simulink model "ICE_assignment"  (R2022a)
settings: Solver=FixedStepDiscrete  StartTime=0.0  StopTime=inf  RelTol=1e-3
undefined symbols (not defined in the file): Friend_Distance, Friend_Latitude, Friend_Longitude, My_Distance, My_Latitude, My_Longitude, sender
libraries: androidcommunicationlib x13, androiduilib x8, androidaudiovideolib x3, androidsensorlib x1
settings Model: Creator=GautamVashishtha  LastModifiedBy=GautamVashishtha
settings OptimizationCC: EnhancedBackFolding=on  PassReuseOutputArgsAs=Individual arguments  ZeroExternalMemoryAtStartup=off  ZeroInternalMemoryAtStartup=off  MaxStackSize=64  OptimizeBlockOrder=speed  DifferentSizesBufferReuse=on  OptimizationCustomize=off  EfficientTunableParamExpr=on
settings DebuggingCC: ParameterTunabilityLossMsg=error
settings HardwareCC: ProdBitPerPointer=32  ProdBitPerSizeT=32  ProdBitPerPtrDiffT=32  ProdLargestAtomicInteger=Long  ProdLargestAtomicFloat=Double  ProdWordSize=32  ProdHWDeviceType=ARM Compatible->ARM Cortex  UseEmbeddedCoderFeatures=off  UseSimulinkCoderFeatures=off
settings SFSimCC: MATLABDynamicMemAlloc=off
settings RTWCC: SystemTargetFile=ert.tlc  HardwareBoard=Android Device  TLCOptions="-aInlineSetEventsForThisBaseRateFcn=TLC_FALSE -aSuppressMultiTaskScheduler=TLC_FALSE  -aRateBasedStepFcn=0"  TemplateMakefile=ert_default_tmf  RTWVerbose=off  Toolchain=Android SDK/NDK Tools
settings CodeAppCC: ForceParamTrailComments=on  IgnoreCustomStorageClasses=off  OperatorAnnotations=on  SimulinkDataObjDesc=on  SFDataObjDesc=on  InsertBlockDesc=on
settings ERTTargetCC: SupportNonInlinedSFcns=on

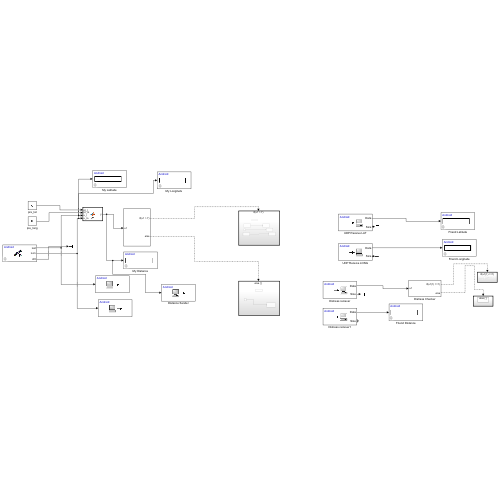
[thumbnail: Simulink's stored preview of the top-level diagram]
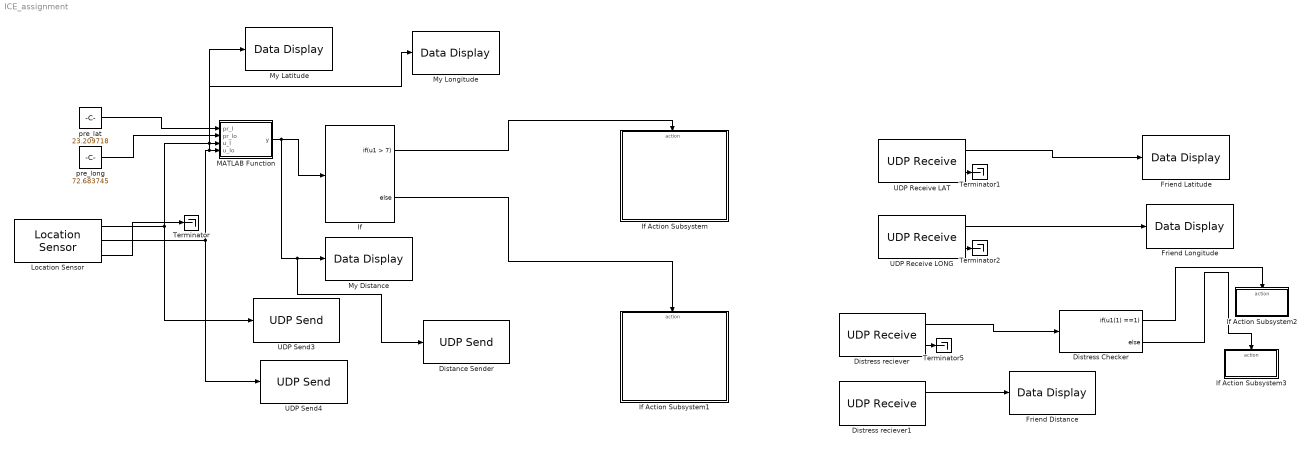
== system ICE_assignment ==
  Distance Sender : androidcommunicationlib/UDP Send  remoteURL='10.7.57.20'  remotePort=1234  localURL='0.0.0.0'  localPortSource=Automatically determine  localPort=-1  sampletime=-1  blockPlatform=Android  separateLengthPort=0
      settings: SourceProductBaseCode=ANDROID
  Distress Checker : If  IfExpression=u1(1) ==1
  Distress reciever : androidcommunicationlib/UDP Receive  localURL='0.0.0.0'  localPort=3000  remoteURL='0.0.0.0'  remotePort=-1  recvBufferSize=8192  signalDatatype=double  dims=1  isVarSize=off  showBlockingTime=off  blockingTime=0  sampletime=0.1  blockPlatform=Android
      settings: SourceProductBaseCode=ANDROID
  Distress reciever1 : androidcommunicationlib/UDP Receive  localURL='0.0.0.0'  localPort=1234  remoteURL='0.0.0.0'  remotePort=-1  recvBufferSize=8192  signalDatatype=double  dims=1  isVarSize=off  showBlockingTime=off  blockingTime=0  sampletime=0.1  blockPlatform=Android
      settings: SourceProductBaseCode=ANDROID
  Friend Distance : androiduilib/Data Display  DataDisplayId=sender/Friend_Distance  Format=Float  Precision=6  SimulateUsing=Code generation  blockPlatform=Android
      settings: SourceProductBaseCode=ANDROID
  Friend Latitude : androiduilib/Data Display  DataDisplayId=sender/Friend_Latitude  Format=Float  Precision=6  SimulateUsing=Code generation  blockPlatform=Android
      settings: SourceProductBaseCode=ANDROID
  Friend Longitude : androiduilib/Data Display  DataDisplayId=sender/Friend_Longitude  Format=Float  Precision=6  SimulateUsing=Code generation  blockPlatform=Android
      settings: SourceProductBaseCode=ANDROID
  If : If  IfExpression=u1 > 7
  If Action Subsystem : Subsystem  TreatAsAtomicUnit=on
  If Action Subsystem1 : Subsystem  TreatAsAtomicUnit=on
  If Action Subsystem2 : Subsystem  TreatAsAtomicUnit=on
  If Action Subsystem3 : Subsystem  TreatAsAtomicUnit=on
  Location Sensor : androidsensorlib/Location Sensor  OutputVector=off  SampleTime=10  BlockPlatform=Android
      settings: SourceProductBaseCode=ANDROID
  MATLAB Function : MATLAB Function  TreatAsAtomicUnit=on
  My Distance : androiduilib/Data Display  DataDisplayId=sender/My_Distance  Format=Float  Precision=6  SimulateUsing=Code generation  blockPlatform=Android
      settings: SourceProductBaseCode=ANDROID
  My Latitude : androiduilib/Data Display  DataDisplayId=sender/My_Latitude  Format=Float  Precision=6  SimulateUsing=Code generation  blockPlatform=Android
      settings: SourceProductBaseCode=ANDROID
  My Longitude : androiduilib/Data Display  DataDisplayId=sender/My_Longitude  Format=Float  Precision=6  SimulateUsing=Code generation  blockPlatform=Android
      settings: SourceProductBaseCode=ANDROID
  Terminator{,1..2,5} (4 alike) : Terminator
  UDP Receive LAT : androidcommunicationlib/UDP Receive  localURL='0.0.0.0'  localPort=5000  remoteURL='0.0.0.0'  remotePort=-1  recvBufferSize=8192  signalDatatype=double  dims=1  isVarSize=off  showBlockingTime=off  blockingTime=0  sampletime=0.1  blockPlatform=Android
      settings: SourceProductBaseCode=ANDROID
  UDP Receive LONG : androidcommunicationlib/UDP Receive  localURL='0.0.0.0'  localPort=4000  remoteURL='0.0.0.0'  remotePort=-1  recvBufferSize=8192  signalDatatype=double  dims=1  isVarSize=off  showBlockingTime=off  blockingTime=0  sampletime=0.1  blockPlatform=Android
      settings: SourceProductBaseCode=ANDROID
  UDP Send3 : androidcommunicationlib/UDP Send  remoteURL='10.7.57.20'  remotePort=5000  localURL='0.0.0.0'  localPortSource=Automatically determine  localPort=-1  sampletime=-1  blockPlatform=Android  separateLengthPort=0
      settings: SourceProductBaseCode=ANDROID
  UDP Send4 : androidcommunicationlib/UDP Send  remoteURL='10.7.57.20'  remotePort=4000  localURL='0.0.0.0'  localPortSource=Automatically determine  localPort=-1  sampletime=-1  blockPlatform=Android  separateLengthPort=0
      settings: SourceProductBaseCode=ANDROID
  pre_lat : Constant  Value=23.209718  SampleTime=0.1
  pre_long : Constant  Value=72.683745  SampleTime=0.1
  wires:
  Location Sensor/2 -> My Longitude/1, MATLAB Function/4(u_lo), UDP Send4/1
  MATLAB Function/1(y) -> Distance Sender/1, My Distance/1, If/1
  Location Sensor/3 -> Terminator/1
  pre_lat/1 -> MATLAB Function/1(pr_l)
  pre_long/1 -> MATLAB Function/2(pr_lo)
  Location Sensor/1 -> My Latitude/1, MATLAB Function/3(u_l), UDP Send3/1
  If/1 -> If Action Subsystem/Action
  If/2 -> If Action Subsystem1/Action
  UDP Receive LONG/1 -> Friend Longitude/1
  Distress reciever/1 -> Distress Checker/1
  Distress reciever/2 -> Terminator5/1
  UDP Receive LAT/1 -> Friend Latitude/1
  UDP Receive LAT/2 -> Terminator1/1
  UDP Receive LONG/2 -> Terminator2/1
  Distress Checker/1 -> If Action Subsystem2/Action
  Distress Checker/2 -> If Action Subsystem3/Action
  Distress reciever1/1 -> Friend Distance/1

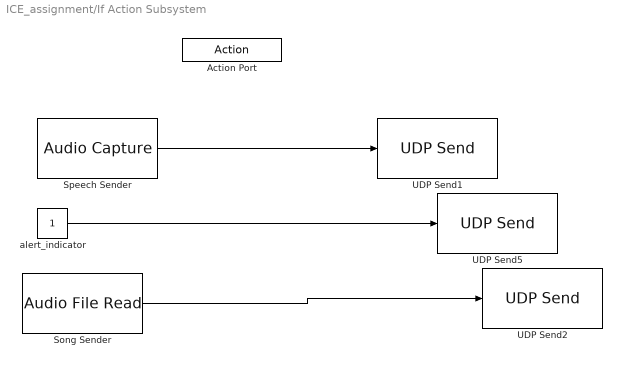
== system ICE_assignment/If Action Subsystem ==
  Action Port : ActionPort  ActionPortLabel=if(u1 > 7)
  Song Sender : androidaudiovideolib/Audio File Read  FileName=guitartune.wav  FrameSize=4410
      settings: SourceProductBaseCode=ANDROID
  Speech Sender : androidaudiovideolib/Audio Capture  SampleFreq=44100  FrameSize=4410  SampleTime=0.1  SimulateUsing=Code generation  DeviceStr=0  QueueDuration=0  BlockPlatform=Android  AudioSamplingFreq=44100
      settings: SourceProductBaseCode=ANDROID
  UDP Send1 : androidcommunicationlib/UDP Send  remoteURL='10.7.57.20'  remotePort=8000  localURL='0.0.0.0'  localPortSource=Automatically determine  localPort=-1  sampletime=-1  blockPlatform=Android  separateLengthPort=0
      settings: SourceProductBaseCode=ANDROID
  UDP Send2 : androidcommunicationlib/UDP Send  remoteURL='10.7.57.20'  remotePort=8001  localURL='0.0.0.0'  localPortSource=Automatically determine  localPort=-1  sampletime=-1  blockPlatform=Android  separateLengthPort=0
      settings: SourceProductBaseCode=ANDROID
  UDP Send5 : androidcommunicationlib/UDP Send  remoteURL='10.7.57.20'  remotePort=3000  localURL='0.0.0.0'  localPortSource=Automatically determine  localPort=-1  sampletime=-1  blockPlatform=Android  separateLengthPort=0
      settings: SourceProductBaseCode=ANDROID
  alert_indicator : Constant
  wires:
  Speech Sender/1 -> UDP Send1/1
  alert_indicator/1 -> UDP Send5/1
  Song Sender/1 -> UDP Send2/1

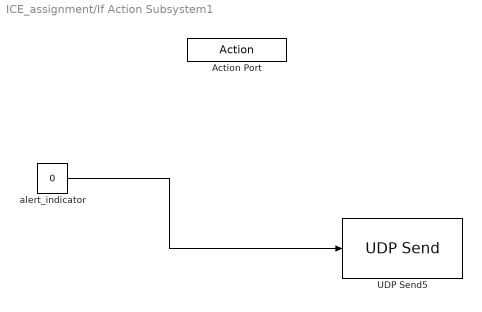
== system ICE_assignment/If Action Subsystem1 ==
  Action Port : ActionPort  ActionPortLabel=else
  UDP Send5 : androidcommunicationlib/UDP Send  remoteURL='10.7.57.20'  remotePort=3000  localURL='0.0.0.0'  localPortSource=Automatically determine  localPort=-1  sampletime=-1  blockPlatform=Android  separateLengthPort=0
      settings: SourceProductBaseCode=ANDROID
  alert_indicator : Constant  Value=0  SampleTime=0.1
  wires:
  alert_indicator/1 -> UDP Send5/1

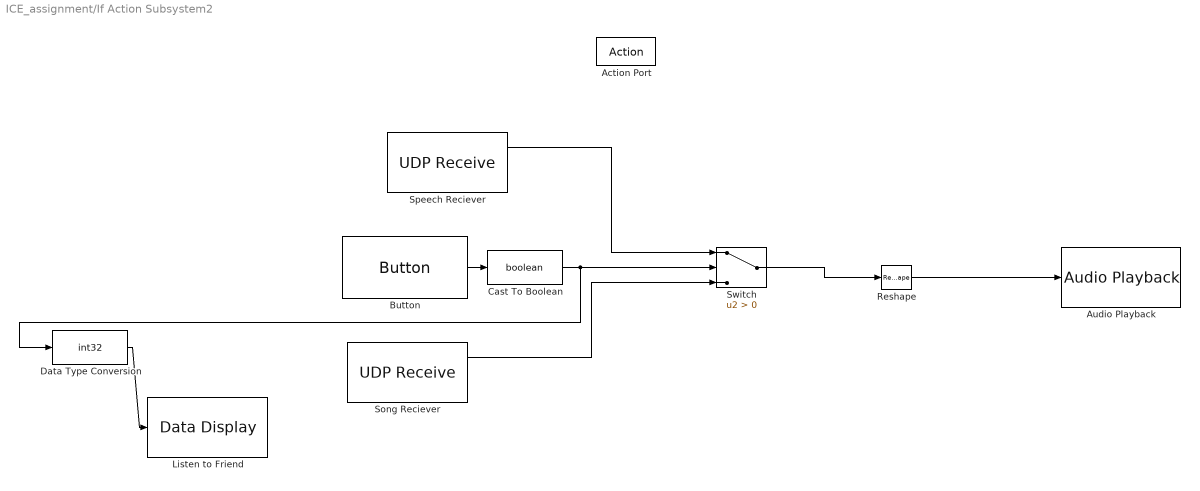
== system ICE_assignment/If Action Subsystem2 ==
  Action Port : ActionPort  ActionPortLabel=if(u1(1) ==1)
  Audio Playback : androidaudiovideolib/Audio Playback  SampleFreq=44100  AudioSamplingFreq=44100  SampleTime=0.1  DeviceStr=0  QueueDuration=0  BlockPlatform=Android
      settings: SourceProductBaseCode=ANDROID
  Button : androiduilib/Button  ButtonState=Not pressed  ButtonId=sender/If_Action_Subsystem2/Button  State=off  SampleTime=0.1  BlockPlatform=Android
      settings: SourceProductBaseCode=ANDROID
  Cast To Boolean : DataTypeConversion  OutDataTypeStr=boolean  SaturateOnIntegerOverflow=off  RndMeth=Floor
  Data Type Conversion : DataTypeConversion  OutDataTypeStr=int32  SaturateOnIntegerOverflow=off  RndMeth=Floor
  Listen to Friend : androiduilib/Data Display  DataDisplayId=sender/If_Action_Subsystem2/Listen_to_Friend  Format=Integer  Precision=6  SimulateUsing=Code generation  blockPlatform=Android
      settings: SourceProductBaseCode=ANDROID
  Reshape : Reshape  OutputDimensionality=Customize  OutputDimensions=[4410,2]
  Song Reciever : androidcommunicationlib/UDP Receive  localURL='0.0.0.0'  localPort=8001  remoteURL='0.0.0.0'  remotePort=-1  recvBufferSize=8192  signalDatatype=int16  dims=8820  isVarSize=off  showBlockingTime=off  blockingTime=0  sampletime=0.1  blockPlatform=Android
      settings: SourceProductBaseCode=ANDROID
  Speech Reciever : androidcommunicationlib/UDP Receive  localURL='0.0.0.0'  localPort=8000  remoteURL='0.0.0.0'  remotePort=-1  recvBufferSize=8192  signalDatatype=int16  dims=8820  isVarSize=off  showBlockingTime=off  blockingTime=0  sampletime=0.1  blockPlatform=Android
      settings: SourceProductBaseCode=ANDROID
  Switch : Switch  Criteria=u2 > Threshold  SaturateOnIntegerOverflow=off  InputSameDT=off
  wires:
  Reshape/1 -> Audio Playback/1
  Button/1 -> Cast To Boolean/1
  Speech Reciever/1 -> Switch/1
  Song Reciever/1 -> Switch/3
  Switch/1 -> Reshape/1
  Data Type Conversion/1 -> Listen to Friend/1
  Cast To Boolean/1 -> Data Type Conversion/1, Switch/2

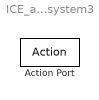
== system ICE_assignment/If Action Subsystem3 ==
  Action Port : ActionPort  ActionPortLabel=else

== matlab function ICE_assignment/MATLAB Function ==
  data: pr_l input; y output; pr_lo input; u_l input; u_lo input
function y = fcn(pr_l,pr_lo,u_l,u_lo)
 dlat = (pr_l-u_l) .* pi / 180;
 dlon = (pr_lo-u_lo).*pi/180;
 lat1 = (pr_l).*pi/180;
 lat2 = (u_l).* pi / 180;
 a = (sin(dlat./2)).^2 + cos(lat1) .* cos(lat2) .* (sin(dlon./2)).^2;
 c = 2 .* asin(sqrt(a));
 c = c*6372.8*1000;
 y = c;
 if (y>10)
     y = 7.8;
 end 
end
